simulink model "algo2"  (R2021a)
settings: Solver=VariableStepAuto  StartTime=0.0  StopTime=1.5  RelTol=1e-3
values from neighbouring files (symbols this model uses):
  b = ball(j)    [ATV7.m]
  k2 = kall(i)    [ATV7.m]
  Xsnub = -0.05    [ATV7.m]
settings Model: Creator=Home  LastModifiedBy=Home

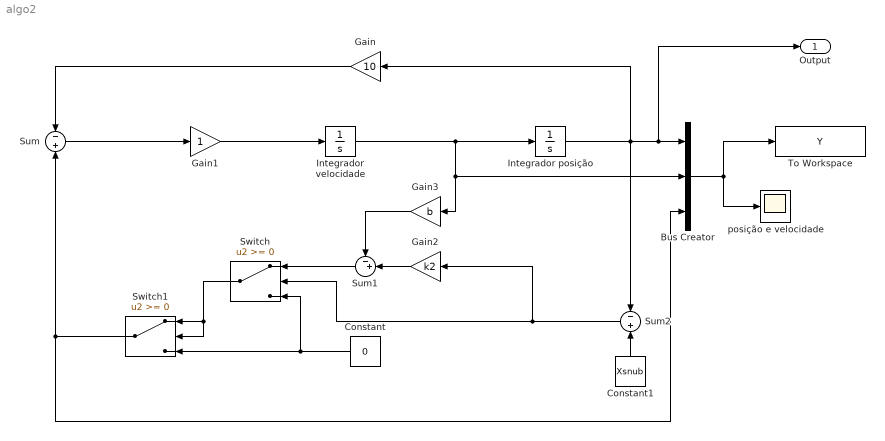
== system algo2 ==
  Bus Creator : BusCreator  Inputs=3
  Constant : Constant  Value=0
  Constant1 : Constant  Value=Xsnub
  Gain : Gain  Gain=10
  Gain1 : Gain
  Gain2 : Gain  Gain=k2
  Gain3 : Gain  Gain=b
  Integrador posição : Integrator  InitialCondition=0.05
  Integrador velocidade : Integrator  InitialCondition=-0.5
  Sum : Sum  Inputs=-|+
  Sum1 : Sum  Inputs=-+|
  Sum2 : Sum  Inputs=-|+
  Switch : Switch
  Switch1 : Switch
  To Workspace : ToWorkspace  VariableName=Y  SampleTime=-1
      settings: Save2DSignal=2-D array (concatenate along first dimension)
  posição e velocidade : Scope
  Output : Outport
  wires:
  Switch1/1 -> Sum/2, Bus Creator/3
  Constant1/1 -> Sum2/2
  Sum/1 -> Gain1/1
  Gain2/1 -> Sum1/2
  Gain/1 -> Sum/1
  Bus Creator/1 -> posição e velocidade/1, To Workspace/1
  Integrador velocidade/1 -> Bus Creator/2, Gain3/1, Integrador posição/1
  Gain3/1 -> Sum1/1
  Gain1/1 -> Integrador velocidade/1
  Integrador posição/1 -> Output/1, Bus Creator/1, Sum2/1, Gain/1
  Sum1/1 -> Switch/1
  Switch/1 -> Switch1/2, Switch1/1
  Constant/1 -> Switch/3, Switch1/3
  Sum2/1 -> Gain2/1, Switch/2
